simulink model "new_Inversor_full_bridge"  (R2015a)
settings: Solver=ode23tb  StartTime=0.0  StopTime=0.1  MaxStep=0.5e-6  RelTol=1e-3
libraries: powerlib x10, simulink x1
settings Model: Creator=Leandro  LastModifiedBy=Iury
settings DataIOCC: SignalLoggingSaveFormat=ModelDataLogs
settings DebuggingCC: UnderspecifiedInitializationDetection=Classic  MergeDetectMultiDrivingBlocksExec=none  MaxConsecutiveZCsMsg=none  SolverPrmCheckMsg=warning  FcnCallInpInsideContextMsg=UseLocalSettings  StateNameClashWarn=warning
settings GRTTargetCC: CombineOutputUpdateFcns=off  GRTInterface=on

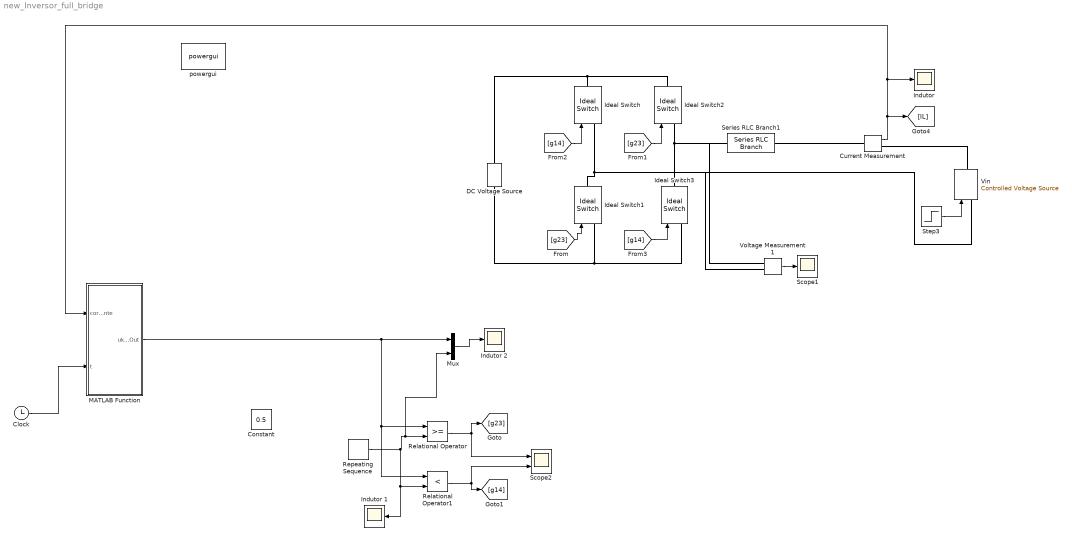
== system new_Inversor_full_bridge ==
  Clock : Clock
  Constant : Constant  Value=0.5
  Current Measurement : powerlib/Measurements/Current Measurement  PhasorSimulation=off  OutputType=Complex  PSBequivalent=0
  DC Voltage Source : powerlib/Electrical Sources/DC Voltage Source  Amplitude=200  Measurements=None
  Ideal Switch{,1..3} (4 alike) : powerlib/Power Electronics/Ideal Switch  Ron=1e-6  Lon=0  IC=0  Rs=1e5  Cs=inf  Measurements=off
  "Indutor " : Scope
      settings: TimeRange=0.05  YMin=0.9  YMax=1.85  SaveName=i
  Indutor 1 : Scope
      settings: TimeRange=0.05  YMin=0  YMax=20  SaveName=i1
  Indutor 2 : Scope
      settings: TimeRange=0.05  YMin=0  YMax=20  SaveName=i2
  MATLAB Function : MATLAB Function  TreatAsAtomicUnit=on
  Mux : Mux  Inputs=2
  Relational Operator : RelationalOperator  OutDataTypeStr=boolean
  Relational Operator1 : RelationalOperator  Operator=<  OutDataTypeStr=boolean
  Repeating Sequence : simulink/Sources/Repeating Sequence  rep_seq_t=[0 1/20000 1/10000]  rep_seq_y=[0 1 0]
  Scope1 : Scope
      settings: TimeRange=0.01
  Scope2 : Scope  NumInputPorts=2
      settings: TimeRange=0.05  YMin=0~0  YMax=1~1  SaveName=ScopeData2
  Series RLC Branch1 : powerlib/Elements/Series RLC Branch  LConnTagsString=__new0  RConnTagsString=__new0  BranchType=R  Resistance=10  Inductance=2e-3  SetiL0=off  InitialCurrent=0  Capacitance=1.0  Setx0=off  InitialVoltage=0  Measurements=None
  Step3 : Step  Time=0  After=0  SampleTime=0
  Vin : powerlib/Electrical Sources/Controlled Voltage Source  Initialize=on  Source_Type=AC  Amplitude=0  Phase=0  Frequency=0  Measurements=None
  Voltage Measurement1 : powerlib/Measurements/Voltage Measurement  PhasorSimulation=off  OutputType=Complex  PSBequivalent=0
  powergui : powerlib/powergui  Priority=1  SimulationMode=Continuous  SolverType=Tustin  SampleTime=50e-6  frequency=60  SPID=on  DisableSnubberDevices=off  DisableRonSwitches=off  DisableVfSwitches=off  SwTol=0  DisplayEquations=off  Interpol=off  methode=off  Ts=0  FunctionMessages=off  echomessages=off  HookPort=off  EnableUseOfTLC=off  x0status=blocks  frequencyindice=0  Pbase=100e6  ErrMax=1e-4  Iterations=50  UnitsV=kV  UnitsW=MW  buscounter=0  RestoreLinks=warning  ResistiveCurrentMeasurement=off  Frange=[0:2:500]  Ylog=off  Xlog=on  ShowGrid=off  save=off  variable=ZData  structure=0  ZoomFFT=off  StartTime=0.0  cycles=1  DisplayStyle=1  fundamental=60  FreqAxis=off  MaxFrequency=1000  frequencyindicesteady=1  RmsSteady=1  display=off
  wires:
  Repeating Sequence/1 -> Indutor 1/1, Relational Operator1/2, Mux/2, Relational Operator/2
  Relational Operator/1 -> [g23], Scope2/1
  Relational Operator1/1 -> [g14], Scope2/2
  [g23] -> Ideal Switch1/1
  [g23] -> Ideal Switch2/1
  [g14] -> Ideal Switch/1
  [g14] -> Ideal Switch3/1
  Current Measurement/1 -> [IL], "Indutor "/1, MATLAB Function/1(corrente)
  Mux/1 -> Indutor 2/1
  Voltage Measurement1/1 -> Scope1/1
  Step3/1 -> Vin/1
  Clock/1 -> MATLAB Function/2(t)
  MATLAB Function/1(ukNextOut) -> Relational Operator1/1, Relational Operator/1, Mux/1
  connections:
  Ideal Switch3/RConn1 -- Voltage Measurement1/LConn1 -- Series RLC Branch1/RConn1 -- Ideal Switch2/LConn1
  Ideal Switch2/RConn1 -- DC Voltage Source/RConn1 -- Ideal Switch/RConn1
  Ideal Switch3/LConn1 -- DC Voltage Source/LConn1 -- Ideal Switch1/LConn1
  Ideal Switch1/RConn1 -- Voltage Measurement1/LConn2 -- Vin/LConn1 -- Ideal Switch/LConn1
  Current Measurement/LConn1 -- Series RLC Branch1/LConn1
  Current Measurement/RConn1 -- Vin/RConn1

== matlab function new_Inversor_full_bridge/MATLAB Function ==
  data: corrente input; t input; ukNextOut output
function ukNextOut = fcn(corrente, t)

k1 = -22.626994881450905;
k2 = -0.561421978901323;
k3 = 79.163345802203452;
k4 = -76.791082664183065;

persistent pontosig;
pontosig = 167;

pi = 3.14159265;
Sd11 = 0.03125;
Sd21 = 0;
Rd11 = 1.998579261776922;
Rd21 = 1;
Rd12 = -0.999999980007103;
Rd22 = 0;

% Variáveis
t_ks = 0;	                  		
n = 0;
pontos_am = 0;
modul_ma_k = 0;
modul_ma_nxt1 = 0;
v_abf_k = 0;
ig_k = 0;
ig_ref_ks=0;
ig_ref_k=0;
Vcc = 200;
ig_ref_nxt2 = 0;
ig_cont_nxt1 = 0;
ig_ref_amost_ks = 0;
v_tri = 0;
sa = 0;
sb = 0;
u_ks=0;
x_ks=0;
theta_ks=0;
rho1_ks=0;
rho2_ks=0;
Rf = 0.1;
Lf = 0.005;
Ig_pk = 10;
theta = 0;
w = 376.99;
u_k=0.5;

persistent u_nxt1;
u_nxt1 = 0.5;

persistent TPER;

rho1_ks_nxt=0;
rho2_ks_nxt=0;
Fs = 10000;
Ts = 1.0e-4;		
Fsw = 10000;
Tsw = 1.0e-4;      
Pontos_fs = 200;  
Pontos_fsw = 200;
persistent t_sample;
t_sample = 200;

ig_ref_k = Ig_pk*sin(w*t);
     
%Controlador
if t_sample == Pontos_fs 
	ig_k = corrente;

	rho1_ks = rho1_ks_nxt;
	rho2_ks = rho2_ks_nxt;
		
    ig_ref_ks = ig_ref_k;
        
    modul_ma_k = modul_ma_nxt1;
    
    u_k = u_nxt1;
   
       
    modul_ma_nxt1 = k1*ig_k + k2*modul_ma_k + k3*rho1_ks + k4*rho2_ks;
    u_nxt1 = (modul_ma_nxt1/(2*Vcc))+0.5;
  
        
   % rho1_ks_nxt = -Sd11*ig_k + 0*modul_ma_k + Rd11*rho1_ks + Rd12*rho2_ks + 0*modul_ma_nxt1 + Sd11 * ig_ref_ks;
    %rho2_ks_nxt = -Sd21*ig_k + 0*modul_ma_k + Rd21*rho1_ks + Rd22*rho2_ks + 0*modul_ma_nxt1 + Sd21 * ig_ref_ks;
        
    x_ks = ig_k;
    t_ks = t_ks + Ts;   
    
end

 %Modulador DSP

    ukNextOut = u_nxt1;
    
    t_sample = t_sample + 1;
end
